simulink model "StablePlant"  (R2017b)
settings: Solver=VariableStepAuto  StartTime=0.0  StopTime=10.0  RelTol=1e-3
values from neighbouring files (symbols this model uses):
  Ts = 0.005    [closed_loop.m]    (also in open_loop.m)
settings Model: Creator=tomas  LastModifiedBy=tomas

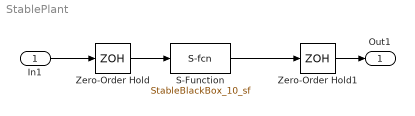
== system StablePlant ==
  In1 : Inport
  S-Function : S-Function  FunctionName=StableBlackBox_10_sf  SFunctionDeploymentMode=off  EnableBusSupport=off
  Zero-Order Hold : ZeroOrderHold  SampleTime=Ts
  Zero-Order Hold1 : ZeroOrderHold  SampleTime=Ts
  Out1 : Outport
  wires:
  S-Function/1 -> Zero-Order Hold1/1
  Zero-Order Hold/1 -> S-Function/1
  In1/1 -> Zero-Order Hold/1
  Zero-Order Hold1/1 -> Out1/1
